simulink model "W2P4"  (R2020b)
settings: Solver=VariableStepAuto  StartTime=0.0  StopTime=5  RelTol=1e-3
undefined symbols (not defined in the file or in its folder): b, J, Ke, Kt, L, R
libraries: pid_lib x1
settings Model: DataDictionary=W2P4_dd.sldd  Creator=saadh  LastModifiedBy=saadh

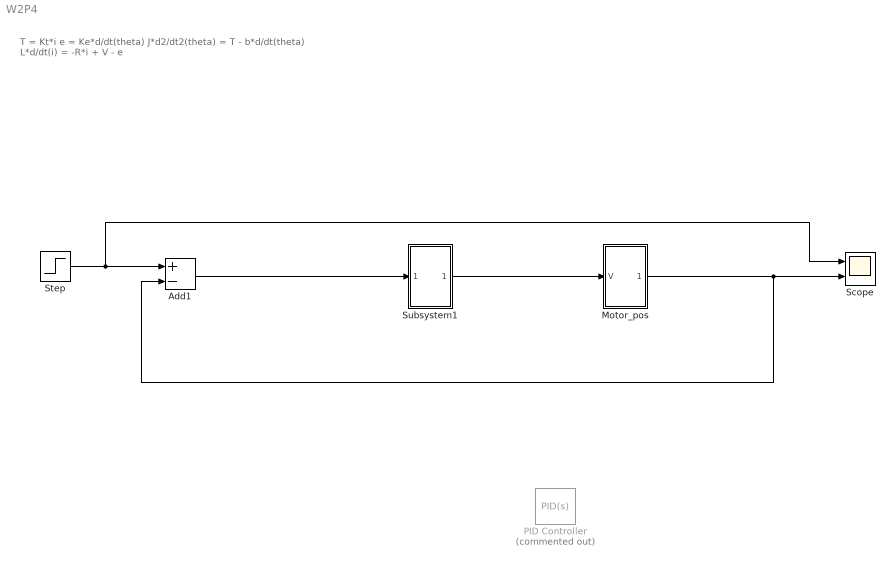
== system W2P4 ==
  note: T = Kt*i
      | e = Ke*d/dt(theta)
      | J*d2/dt2(theta) = T - b*d/dt(theta)
      | L*d/dt(i) = -R*i + V - e
  Add1 : Sum  Inputs=+-
  Motor_pos : Subsystem
  PID Controller : pid_lib/PID Controller  Commented=on  Controller=PID  Form=Parallel  TimeDomain=Continuous-time  UseExternalTs=off  SampleTime=-1  IntegratorMethod=Forward Euler  FilterMethod=Forward Euler  ControllerParametersSource=internal  P=18.8618161296239  I=554.412400621923  D=0.154124143680084  UseFilter=on  N=1893.60660908492  TunerSelectOption=Transfer Function Based (PID Tuner App)  InitialConditionSource=internal  InitialConditionForIntegrator=0  InitialConditionForFilter=0  DifferentiatorICPrevScaledInput=0  ExternalReset=none  TrackingMode=off  Kt=1  LimitOutput=off  SatLimitsSource=internal  UpperSaturationLimit=inf  LowerSaturationLimit=-inf  LinearizeAsGain=on  AntiWindupMode=none  Kb=1  POutMin=[]  POutMax=[]  IOutMin=[]  IOutMax=[]  DOutMin=[]  DOutMax=[]  NOutMin=[]  NOutMax=[]  SumOutMin=[]  SumOutMax=[]  SaturationOutMin=[]  SaturationOutMax=[]  PParamMin=[]  PParamMax=[]  IParamMin=[]  IParamMax=[]  DParamMin=[]  DParamMax=[]  NParamMin=[]  NParamMax=[]  KbParamMin=[]  KbParamMax=[]  KtParamMin=[]  KtParamMax=[]  KbOutMin=[]  KbOutMax=[]  KtOutMin=[]  KtOutMax=[]  IntegratorOutMin=[]  IntegratorOutMax=[]  FilterOutMin=[]  FilterOutMax=[]  SumI1OutMin=[]  SumI1OutMax=[]  SumI2OutMin=[]  SumI2OutMax=[]  SumI3OutMin=[]  SumI3OutMax=[]  SumI4OutMin=[]  SumI4OutMax=[]  SumDOutMin=[]  SumDOutMax=[]  DifferentiatorOutMin=[]  DifferentiatorOutMax=[]  FilterDiffOutCoefMin=[]  FilterDiffOutCoefMax=[]  ReciprocalOutMin=[]  ReciprocalOutMax=[]  SumDenOutMin=[]  SumDenOutMax=[]  SumNumOutMin=[]  SumNumOutMax=[]  DivideOutMin=[]  DivideOutMax=[]  UdiffTsProdOutMin=[]  UdiffTsProdOutMax=[]  NTsProdOutMin=[]  NTsProdOutMax=[]  UintegralTsProdOutMin=[]  UintegralTsProdOutMax=[]  UngainTsProdOutMin=[]  UngainTsProdOutMax=[]  IntegratorContinuousStateAttributes=''  IntegratorStateMustResolveToSignalObject=off  IntegratorRTWStateStorageClass=Auto  FilterContinuousStateAttributes=''  FilterStateMustResolveToSignalObject=off  FilterRTWStateStorageClass=Auto  ParallelPVariant=InternalParameters  IdealPVariant=Disabled  IVariant=InternalParameters  DVariant=InternalParameters  IntegratorVariant=Continuous  SatVariant=Disabled  AWVariant=Passthrough  PCopyVariant=Disabled  TRVariant=Disabled  FdbkBlocksVariant=Forward  IdealPFdbkVariant=Disabled  SatFdbkVariant=Disabled  DerivativeFilterVariant=ContFilter  NVariant=InternalParameters  NCopyVariant=Disabled  FilterICVariant=InternalICsFilter  IntegratorICVariant=InternalICs  ExternalResetVariant=Disabled  TRSumVariant=Passthrough  SumFdbkVariant=Disabled  SumVariant=Sum_PID  TsampFilterVariant=InternalTs  TsampNgainVariant=Passthrough  TsampIntegralVariant=Passthrough  ExternalSaturationOutDataTypeStr=Inherit: Same as second input
  Scope : Scope  NumInputPorts=2
  Step : Step  SampleTime=0
  Subsystem1 : ModelReference  ModelNameDialog=Subsystem1  SimulationMode=Normal  ModelReferenceVersion=1.3
  wires:
  Step/1 -> Scope/1, Add1/1
  Motor_pos/1(theta) -> Add1/2, Scope/2
  Add1/1 -> Subsystem1/1
  Subsystem1/1 -> Motor_pos/1(V)

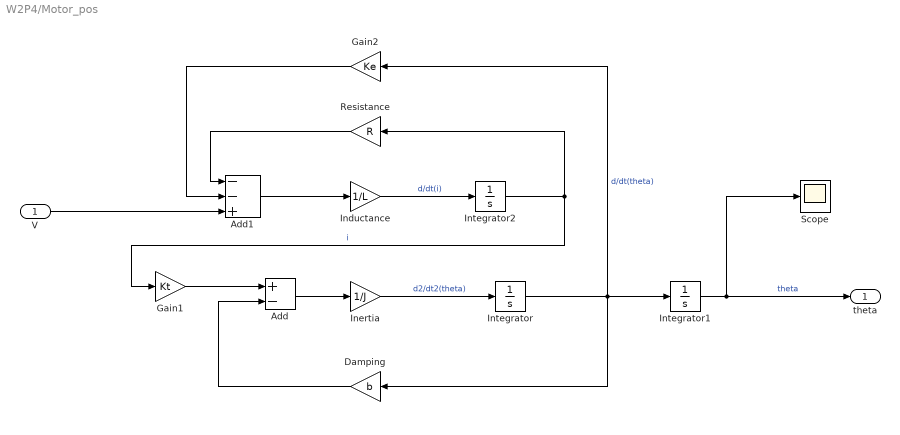
== system W2P4/Motor_pos ==
  V : Inport
  "Add " : Sum  Inputs=+-
  "Add1 " : Sum  Inputs=--+
  Damping : Gain  Gain=b
  Gain1 : Gain  Gain=Kt
  Gain2 : Gain  Gain=Ke
  Inductance : Gain  Gain=1/L
  Inertia : Gain  Gain=1/J
  "Integrator " : Integrator
  "Integrator1 " : Integrator
  "Integrator2 " : Integrator
  Resistance : Gain  Gain=R
  Scope : Scope
  theta : Outport
  wires:
  "Integrator1 "/1 -> theta/1, Scope/1  "theta"
  Gain1/1 -> "Add "/1
  Inductance/1 -> "Integrator2 "/1  "d/dt(i)"
  "Integrator2 "/1 -> Resistance/1, Gain1/1  "i"
  "Add "/1 -> Inertia/1
  "Integrator "/1 -> Gain2/1, Damping/1, "Integrator1 "/1  "d/dt(theta)"
  V/1 -> "Add1 "/3
  Damping/1 -> "Add "/2
  Resistance/1 -> "Add1 "/1
  Inertia/1 -> "Integrator "/1  "d2/dt2(theta)"
  Gain2/1 -> "Add1 "/2
  "Add1 "/1 -> Inductance/1
